simulink model "Horno_LT512_simulink"  (R2023b)
settings: Solver=VariableStepAuto  StartTime=0.0  StopTime=450.0  RelTol=1e-3
settings Model: Creator=Manu  LastModifiedBy=Plantita
settings DebuggingCC: UnconnectedInputMsg=warning  UnconnectedOutputMsg=warning  UnconnectedLineMsg=warning
settings ModelReferenceCC: EnableRefExpFcnMdlSchedulingChecks=on
settings RTWCC: DLArmComputeVersion=19.05

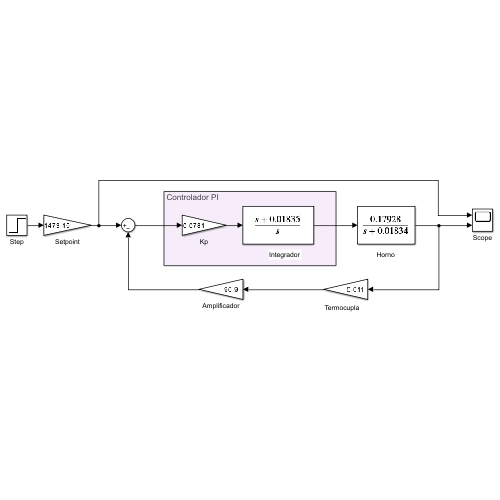
[thumbnail: Simulink's stored preview of the top-level diagram]
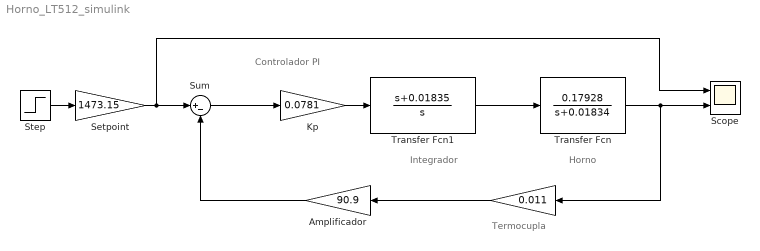
== system Horno_LT512_simulink ==
  note: Integrador
  note: Controlador PI
  note: Termocupla
  note: Horno
  " " : Gain  Gain=0.011
  Amplificador : Gain  Gain=90.9
  Kp : Gain  Gain=0.0781
  Scope : Scope  NumInputPorts=2
  Setpoint : Gain  Gain=1473.15
  Step : Step  SampleTime=0
  Sum : Sum  Inputs=|+-
  Transfer Fcn : TransferFcn  Numerator=[0.17928]  Denominator=[1 0.01834]
  Transfer Fcn1 : TransferFcn  Numerator=[1 0.01835]  Denominator=[1 0]
  wires:
  Transfer Fcn1/1 -> Transfer Fcn/1
  Amplificador/1 -> Sum/2
  " "/1 -> Amplificador/1
  Transfer Fcn/1 -> " "/1, Scope/2
  Step/1 -> Setpoint/1
  Setpoint/1 -> Scope/1, Sum/1
  Kp/1 -> Transfer Fcn1/1
  Sum/1 -> Kp/1
